simulink model "controladorPaola"  (R2023b)
settings: Solver=ode23t  StartTime=0.0  StopTime=60  MaxStep=1e-3  RelTol=1e-3
values from neighbouring files (symbols this model uses):
  AL = double(subs(A_par))    [ANTImodeloMATEMATICOFINAL.m]
  BL = double(subs(B_par))    [ANTImodeloMATEMATICOFINAL.m]
  Blo = 8.18575752786119e-06    (= 8.18575752786e-06)    [ANTImodeloMATEMATICOFINAL.m]
  Bmo = 2.02156082362446e-07    (= 2.02156082362e-07)    [ANTImodeloMATEMATICOFINAL.m]
  CL = double(subs(C_par))    [ANTImodeloMATEMATICOFINAL.m]
  DL = double(subs(D_par))    [ANTImodeloMATEMATICOFINAL.m]
  do = 0.06862-0.021    (= 0.04762)    [ANTImodeloMATEMATICOFINAL.m]
  go = 9.81    [ANTImodeloMATEMATICOFINAL.m]
  Jlo = 0.00100697016255642    (= 0.00100697016256)    [ANTImodeloMATEMATICOFINAL.m]
  Jmo = 2.08549279330578e-07    (= 2.08549279331e-07)    [ANTImodeloMATEMATICOFINAL.m]
  Kes = K(:,1:n)    [ANTImodeloMATEMATICOFINAL.m]
  Ki = -K(:,n+1:end)    [ANTImodeloMATEMATICOFINAL.m]
  Kio = 0.00119530882984502    (= 0.00119530882985)    [ANTImodeloMATEMATICOFINAL.m]
  Kvo = 0.0035694528924319    (= 0.00356945289243)    [ANTImodeloMATEMATICOFINAL.m]
  Lo = 0.667669785204658    (= 0.667669785205)    [ANTImodeloMATEMATICOFINAL.m]
  mo = 0.17244    [ANTImodeloMATEMATICOFINAL.m]
  no = 120    [ANTImodeloMATEMATICOFINAL.m]
  Ro = 5.15610211779038    (= 5.15610211779)    [ANTImodeloMATEMATICOFINAL.m]
  Tm = 0.03    [ANTImodeloMATEMATICOFINAL.m]
  Vin0 = Ro*X10    (= 0)    [ANTImodeloMATEMATICOFINAL.m]
  X10 = 0    [ANTImodeloMATEMATICOFINAL.m]
  X20 = 0    [ANTImodeloMATEMATICOFINAL.m]
  X30 = 0    [ANTImodeloMATEMATICOFINAL.m]
undefined symbols (not defined in the file or in its folder): Ac_2, Bc_2, Cc_2, Dc_2, L, magnitude, sys_d2
libraries: cstblocks x6, slpidlib x4, simulink x4
(part 1 of 2)
settings Model: Creator=hubertdelgado  LastModifiedBy=electronica
settings DebuggingCC: UnconnectedInputMsg=warning  UnconnectedOutputMsg=warning  UnconnectedLineMsg=warning
settings ModelReferenceCC: EnableRefExpFcnMdlSchedulingChecks=on
settings RTWCC: DLArmComputeVersion=19.05

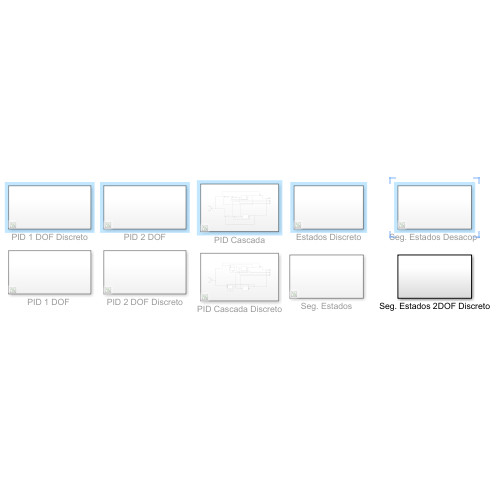
[thumbnail: Simulink's stored preview of the top-level diagram]
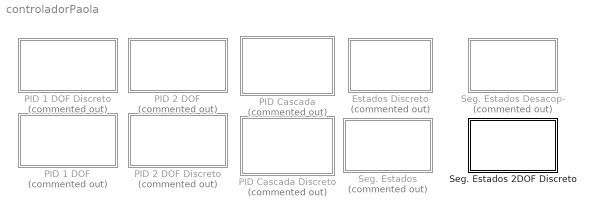
== system controladorPaola ==
  Estados Discreto : Subsystem  Commented=on
  "PID 1 DOF " : Subsystem  Commented=on
  PID 1 DOF Discreto : Subsystem  Commented=on
  PID 2 DOF : Subsystem  Commented=on
  PID 2 DOF Discreto : Subsystem  Commented=on
  PID Cascada : Subsystem  Commented=on
  PID Cascada Discreto : Subsystem  Commented=on
  Seg. Estados : Subsystem  Commented=on
  Seg. Estados 2DOF Discreto : Subsystem
  Seg. Estados Desacop- : Subsystem  Commented=on

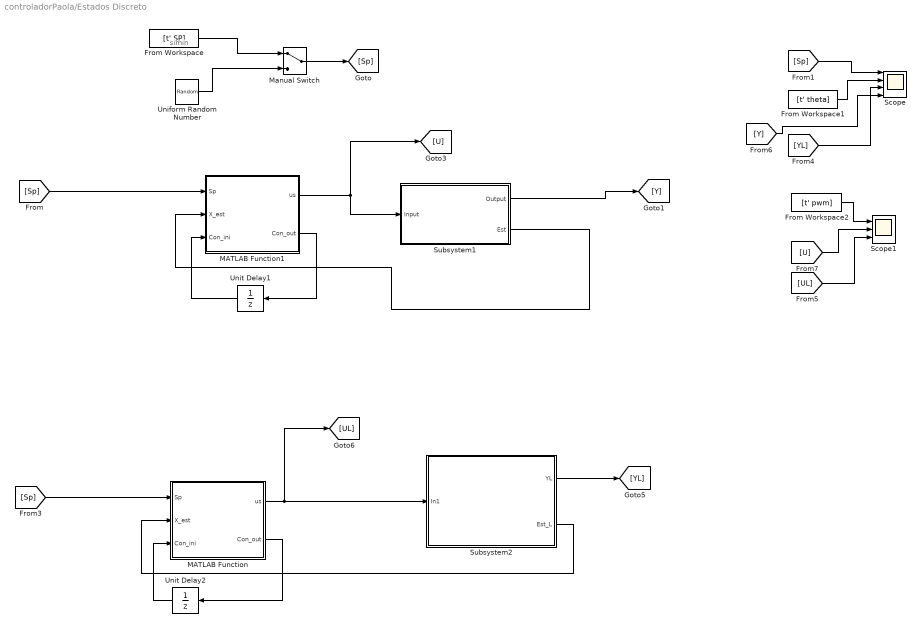
== system controladorPaola/Estados Discreto ==
  note: simin
  From Workspace : FromWorkspace  VariableName=[t' SP]
  From Workspace1 : FromWorkspace  VariableName=[t' theta]
  From Workspace2 : FromWorkspace  VariableName=[t' pwm]
  MATLAB Function : MATLAB Function  TreatAsAtomicUnit=on
  MATLAB Function1 : MATLAB Function  TreatAsAtomicUnit=on
  Manual Switch : ManualSwitch
  Scope : Scope  NumInputPorts=4
  Scope1 : Scope  NumInputPorts=3
  Subsystem1 : Subsystem
  Subsystem2 : Subsystem
  Uniform Random Number : UniformRandomNumber  Minimum=-120*(pi/180)  Maximum=120*(pi/180)  SampleTime=10
  Unit Delay1 : UnitDelay  InitialCondition=zeros(1,2)  SampleTime=Tm  HasFrameUpgradeWarning=on
  Unit Delay2 : UnitDelay  InitialCondition=zeros(1,2)  SampleTime=Tm  HasFrameUpgradeWarning=on
  wires:
  Subsystem1/1(Output) -> [Y]
  MATLAB Function/1(us) -> Subsystem2/1(In1), [UL]
  [Sp] -> MATLAB Function/1(Sp)
  MATLAB Function/2(Con_out) -> Unit Delay2/1
  Unit Delay2/1 -> MATLAB Function/3(Con_ini)
  Subsystem2/2(Est_L) -> MATLAB Function/2(X_est)
  Subsystem2/1(YL) -> [YL]
  Manual Switch/1 -> [Sp]
  [Y] -> Scope/4
  From Workspace2/1 -> Scope1/1
  From Workspace/1 -> Manual Switch/1
  From Workspace1/1 -> Scope/2
  Uniform Random Number/1 -> Manual Switch/2
  [Sp] -> Scope/1
  [UL] -> Scope1/3
  [U] -> Scope1/2
  [YL] -> Scope/3
  Subsystem1/2(Est) -> MATLAB Function1/2(X_est)
  Unit Delay1/1 -> MATLAB Function1/3(Con_ini)
  MATLAB Function1/2(Con_out) -> Unit Delay1/1
  [Sp] -> MATLAB Function1/1(Sp)
  MATLAB Function1/1(us) -> [U], Subsystem1/1(Input)

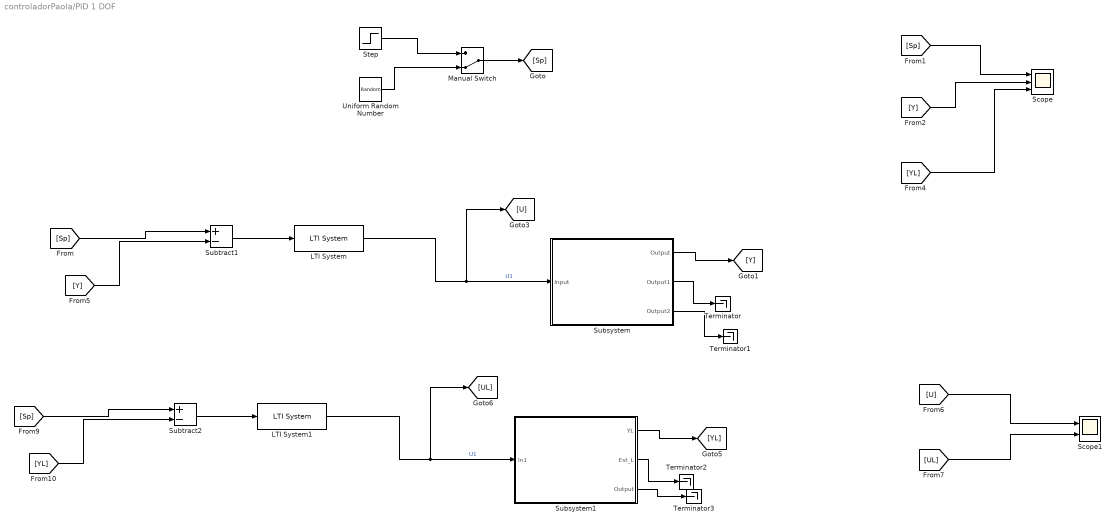
== system controladorPaola/PID 1 DOF  ==
  LTI System : cstblocks/LTI System  sys=Cpids  IC=[]
  LTI System1 : cstblocks/LTI System  sys=Cpids  IC=[]
  Manual Switch : ManualSwitch  CurrentSetting=0
  Scope : Scope  NumInputPorts=3
  Scope1 : Scope  NumInputPorts=2
  Step : Step  Time=0  After=0  SampleTime=0
  Subsystem : Subsystem
  Subsystem1 : Subsystem
  Subtract1 : Sum  Inputs=+-
  Subtract2 : Sum  Inputs=+-
  Terminator{,1..3} (4 alike) : Terminator
  Uniform Random Number : UniformRandomNumber  Minimum=-70*(pi/180)  Maximum=70*(pi/180)  SampleTime=10
  wires:
  Manual Switch/1 -> [Sp]
  Uniform Random Number/1 -> Manual Switch/2
  [U] -> Scope1/1
  [UL] -> Scope1/2
  Step/1 -> Manual Switch/1
  Subtract1/1 -> LTI System/1
  LTI System/1 -> Subsystem/1(Input), [U]  "U1"
  [Sp] -> Subtract1/1
  [Y] -> Subtract1/2
  Subsystem/1(Output) -> [Y]
  Subtract2/1 -> LTI System1/1
  [YL] -> Subtract2/2
  LTI System1/1 -> Subsystem1/1(In1), [UL]  "U1"
  Subsystem1/2(Est_L) -> Terminator2/1
  Subsystem1/1(YL) -> [YL]
  [Sp] -> Subtract2/1
  [Sp] -> Scope/1
  [Y] -> Scope/2
  [YL] -> Scope/3
  Subsystem/2(Output1) -> Terminator/1
  Subsystem/3(Output2) -> Terminator1/1
  Subsystem1/3(Output) -> Terminator3/1

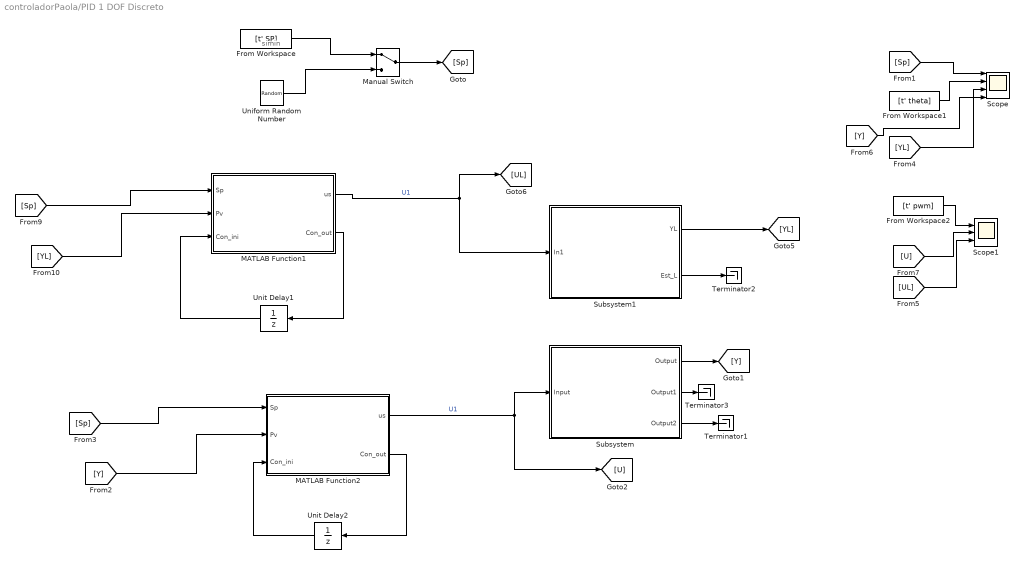
== system controladorPaola/PID 1 DOF Discreto ==
  note: simin
  From Workspace : FromWorkspace  VariableName=[t' SP]
  From Workspace1 : FromWorkspace  VariableName=[t' theta]
  From Workspace2 : FromWorkspace  VariableName=[t' pwm]
  MATLAB Function1 : MATLAB Function  TreatAsAtomicUnit=on
  MATLAB Function2 : MATLAB Function  TreatAsAtomicUnit=on
  Manual Switch : ManualSwitch
  Scope : Scope  NumInputPorts=4
  Scope1 : Scope  NumInputPorts=3
  Subsystem : Subsystem
  Subsystem1 : Subsystem
  Terminator1 : Terminator
  Terminator2 : Terminator
  Terminator3 : Terminator
  Uniform Random Number : UniformRandomNumber  Minimum=-60*(pi/180)  Maximum=60*(pi/180)  SampleTime=10
  Unit Delay1 : UnitDelay  InitialCondition=zeros(4,1)  SampleTime=Tm  HasFrameUpgradeWarning=on
  Unit Delay2 : UnitDelay  InitialCondition=zeros(5,1)  SampleTime=Tm  HasFrameUpgradeWarning=on
  wires:
  Manual Switch/1 -> [Sp]
  Uniform Random Number/1 -> Manual Switch/2
  From Workspace2/1 -> Scope1/1
  [U] -> Scope1/2
  From Workspace/1 -> Manual Switch/1
  [YL] -> MATLAB Function1/2(Pv)
  MATLAB Function1/1(us) -> Subsystem1/1(In1), [UL]  "U1"
  Subsystem1/2(Est_L) -> Terminator2/1
  Subsystem1/1(YL) -> [YL]
  [Sp] -> Scope/1
  From Workspace1/1 -> Scope/2
  [YL] -> Scope/3
  Unit Delay1/1 -> MATLAB Function1/3(Con_ini)
  [Sp] -> MATLAB Function1/1(Sp)
  MATLAB Function1/2(Con_out) -> Unit Delay1/1
  Unit Delay2/1 -> MATLAB Function2/3(Con_ini)
  MATLAB Function2/2(Con_out) -> Unit Delay2/1
  MATLAB Function2/1(us) -> [U], Subsystem/1(Input)  "U1"
  [Sp] -> MATLAB Function2/1(Sp)
  [Y] -> MATLAB Function2/2(Pv)
  Subsystem/1(Output) -> [Y]
  Subsystem/3(Output2) -> Terminator1/1
  Subsystem/2(Output1) -> Terminator3/1
  [UL] -> Scope1/3
  [Y] -> Scope/4

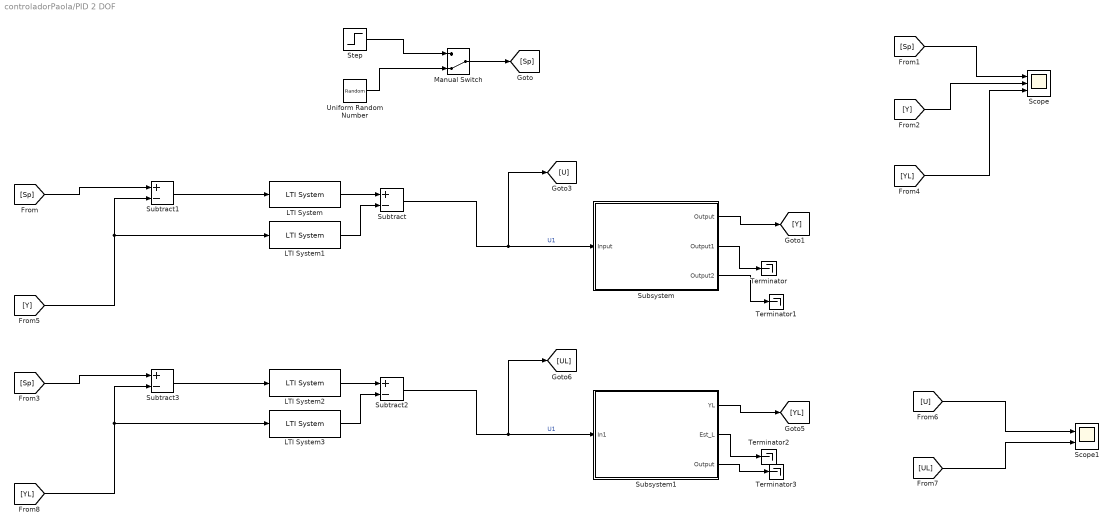
== system controladorPaola/PID 2 DOF ==
  LTI System : cstblocks/LTI System  sys=C1s  IC=[]  PadeOrder=0
  LTI System1 : cstblocks/LTI System  sys=C2s  IC=[]  PadeOrder=0
  LTI System2 : cstblocks/LTI System  sys=C1s  IC=[]  PadeOrder=0
  LTI System3 : cstblocks/LTI System  sys=C2s  IC=[]  PadeOrder=0
  Manual Switch : ManualSwitch  CurrentSetting=0
  Scope : Scope  NumInputPorts=3
  Scope1 : Scope  NumInputPorts=2
  Step : Step  Time=0  After=0  SampleTime=0
  Subsystem : Subsystem
  Subsystem1 : Subsystem
  Subtract{,1..3} (4 alike) : Sum  Inputs=+-
  Terminator{,1..3} (4 alike) : Terminator
  Uniform Random Number : UniformRandomNumber  Minimum=-60*(pi/180)  Maximum=60*(pi/180)  SampleTime=10
  wires:
  LTI System/1 -> Subtract/1
  Subtract1/1 -> LTI System/1
  [Sp] -> Subtract1/1
  [Y] -> LTI System1/1, Subtract1/2
  LTI System1/1 -> Subtract/2
  Subtract2/1 -> Subsystem1/1(In1), [UL]  "U1"
  Subsystem1/3(Output) -> Terminator3/1
  Subtract/1 -> Subsystem/1(Input), [U]  "U1"
  Subsystem1/2(Est_L) -> Terminator2/1
  Subsystem/3(Output2) -> Terminator1/1
  Subsystem1/1(YL) -> [YL]
  Subsystem/2(Output1) -> Terminator/1
  Subsystem/1(Output) -> [Y]
  [Sp] -> Subtract3/1
  LTI System3/1 -> Subtract2/2
  LTI System2/1 -> Subtract2/1
  Subtract3/1 -> LTI System2/1
  [YL] -> LTI System3/1, Subtract3/2
  [UL] -> Scope1/2
  Step/1 -> Manual Switch/1
  Manual Switch/1 -> [Sp]
  [Y] -> Scope/2
  [Sp] -> Scope/1
  [YL] -> Scope/3
  [U] -> Scope1/1
  Uniform Random Number/1 -> Manual Switch/2

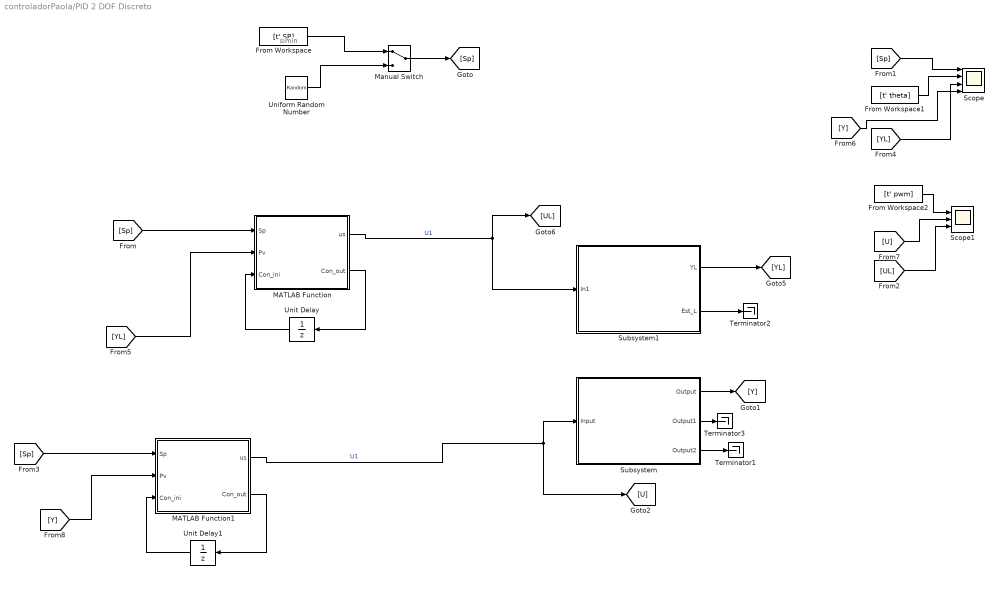
== system controladorPaola/PID 2 DOF Discreto ==
  note: simin
  From Workspace : FromWorkspace  VariableName=[t' SP]
  From Workspace1 : FromWorkspace  VariableName=[t' theta]
  From Workspace2 : FromWorkspace  VariableName=[t' pwm]
  MATLAB Function : MATLAB Function  TreatAsAtomicUnit=on
  MATLAB Function1 : MATLAB Function  TreatAsAtomicUnit=on
  Manual Switch : ManualSwitch
  Scope : Scope  NumInputPorts=4
  Scope1 : Scope  NumInputPorts=3
  Subsystem : Subsystem
  Subsystem1 : Subsystem
  Terminator1 : Terminator
  Terminator2 : Terminator
  Terminator3 : Terminator
  Uniform Random Number : UniformRandomNumber  Minimum=-65*(pi/180)  Maximum=65*(pi/180)  SampleTime=10
  Unit Delay : UnitDelay  InitialCondition=zeros(6,1)  SampleTime=Tm  HasFrameUpgradeWarning=on
  Unit Delay1 : UnitDelay  InitialCondition=zeros(6,1)  SampleTime=Tm  HasFrameUpgradeWarning=on
  wires:
  [Sp] -> MATLAB Function/1(Sp)
  Unit Delay/1 -> MATLAB Function/3(Con_ini)
  MATLAB Function/2(Con_out) -> Unit Delay/1
  From Workspace1/1 -> Scope/2
  [YL] -> Scope/3
  [UL] -> Scope1/3
  [U] -> Scope1/2
  [Sp] -> Scope/1
  Uniform Random Number/1 -> Manual Switch/2
  From Workspace/1 -> Manual Switch/1
  From Workspace2/1 -> Scope1/1
  Manual Switch/1 -> [Sp]
  [Y] -> Scope/4
  Subsystem/2(Output1) -> Terminator3/1
  MATLAB Function/1(us) -> Subsystem1/1(In1), [UL]  "U1"
  Subsystem1/2(Est_L) -> Terminator2/1
  Subsystem1/1(YL) -> [YL]
  Subsystem/3(Output2) -> Terminator1/1
  Subsystem/1(Output) -> [Y]
  MATLAB Function1/1(us) -> [U], Subsystem/1(Input)  "U1"
  [Sp] -> MATLAB Function1/1(Sp)
  Unit Delay1/1 -> MATLAB Function1/3(Con_ini)
  MATLAB Function1/2(Con_out) -> Unit Delay1/1
  [YL] -> MATLAB Function/2(Pv)
  [Y] -> MATLAB Function1/2(Pv)

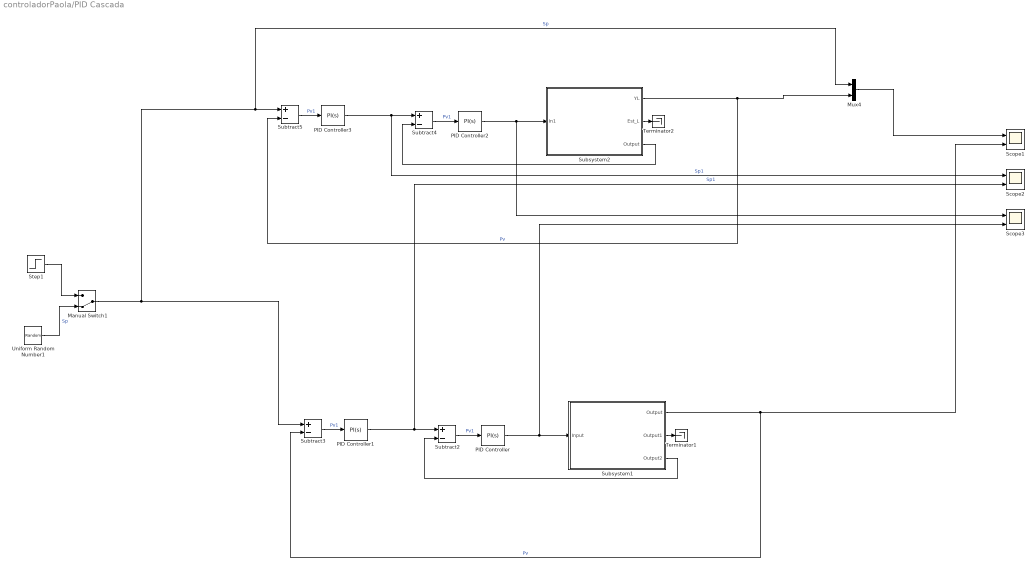
== system controladorPaola/PID Cascada ==
  Manual Switch1 : ManualSwitch  CurrentSetting=0
  Mux4 : Mux  Inputs=2
  PID Controller : slpidlib/PID Controller  Controller=PI  Form=Parallel  TimeDomain=Continuous-time  UseExternalTs=off  SampleTime=-1  IntegratorMethod=Forward Euler  FilterMethod=Forward Euler  ControllerParametersSource=internal  P=0.439531738224972  I=0.0931065859182185  D=35.8399189335653  UseFilter=on  N=15672.9006565225  TunerSelectOption=Transfer Function Based (PID Tuner App)  InitialConditionSource=internal  InitialConditionForIntegrator=0  InitialConditionForFilter=0  DifferentiatorICPrevScaledInput=0  ExternalReset=none  TrackingMode=off  Kt=1  LimitOutput=on  SatLimitsSource=internal  UpperSaturationLimit=100  LowerSaturationLimit=-100  LinearizeAsGain=on  AntiWindupMode=none  Kb=1  POutMin=[]  POutMax=[]  IOutMin=[]  IOutMax=[]  DOutMin=[]  DOutMax=[]  NOutMin=[]  NOutMax=[]  SumOutMin=[]  SumOutMax=[]  SaturationOutMin=[]  SaturationOutMax=[]  PParamMin=[]  PParamMax=[]  IParamMin=[]  IParamMax=[]  DParamMin=[]  DParamMax=[]  NParamMin=[]  NParamMax=[]  KbParamMin=[]  KbParamMax=[]  KtParamMin=[]  KtParamMax=[]  KbOutMin=[]  KbOutMax=[]  KtOutMin=[]  KtOutMax=[]  IntegratorOutMin=[]  IntegratorOutMax=[]  FilterOutMin=[]  FilterOutMax=[]  SumI1OutMin=[]  SumI1OutMax=[]  SumI2OutMin=[]  SumI2OutMax=[]  SumI3OutMin=[]  SumI3OutMax=[]  SumI4OutMin=[]  SumI4OutMax=[]  SumDOutMin=[]  SumDOutMax=[]  DifferentiatorOutMin=[]  DifferentiatorOutMax=[]  FilterDiffOutCoefMin=[]  FilterDiffOutCoefMax=[]  ReciprocalOutMin=[]  ReciprocalOutMax=[]  SumDenOutMin=[]  SumDenOutMax=[]  SumNumOutMin=[]  SumNumOutMax=[]  DivideOutMin=[]  DivideOutMax=[]  UdiffTsProdOutMin=[]  UdiffTsProdOutMax=[]  NTsProdOutMin=[]  NTsProdOutMax=[]  UintegralTsProdOutMin=[]  UintegralTsProdOutMax=[]  UngainTsProdOutMin=[]  UngainTsProdOutMax=[]  IntegratorContinuousStateAttributes=''  IntegratorStateMustResolveToSignalObject=off  IntegratorRTWStateStorageClass=Auto  FilterContinuousStateAttributes=''  FilterStateMustResolveToSignalObject=off  FilterRTWStateStorageClass=Auto  ParallelPVariant=InternalParameters  IdealPVariant=Disabled  IVariant=InternalParameters  DVariant=Disabled  IntegratorVariant=Continuous  SatVariant=Enabled  AWVariant=Passthrough  PCopyVariant=Disabled  TRVariant=Disabled  FdbkBlocksVariant=Forward  IdealPFdbkVariant=Disabled  SatFdbkVariant=Disabled  DerivativeFilterVariant=Disabled  NVariant=Disabled  NCopyVariant=Disabled_SignalSpec  FilterICVariant=Disabled  IntegratorICVariant=InternalICs  ExternalResetVariant=Disabled  TRSumVariant=Passthrough  SumFdbkVariant=Disabled  SumVariant=Sum_PI  TsampFilterVariant=InternalTs  TsampNgainVariant=Passthrough  TsampIntegralVariant=Passthrough  ExternalSaturationOutDataTypeStr=Inherit: Same as second input
  PID Controller1 : slpidlib/PID Controller  Controller=PI  Form=Parallel  TimeDomain=Continuous-time  UseExternalTs=off  SampleTime=-1  IntegratorMethod=Forward Euler  FilterMethod=Forward Euler  ControllerParametersSource=internal  P=0  I=93.1384599522807  D=0.271518816024789  UseFilter=on  N=3961.125137588  TunerSelectOption=Transfer Function Based (PID Tuner App)  InitialConditionSource=internal  InitialConditionForIntegrator=0  InitialConditionForFilter=0  DifferentiatorICPrevScaledInput=0  ExternalReset=none  TrackingMode=off  Kt=1  LimitOutput=on  SatLimitsSource=internal  UpperSaturationLimit=40  LowerSaturationLimit=-40  LinearizeAsGain=on  AntiWindupMode=none  Kb=1  POutMin=[]  POutMax=[]  IOutMin=[]  IOutMax=[]  DOutMin=[]  DOutMax=[]  NOutMin=[]  NOutMax=[]  SumOutMin=[]  SumOutMax=[]  SaturationOutMin=[]  SaturationOutMax=[]  PParamMin=[]  PParamMax=[]  IParamMin=[]  IParamMax=[]  DParamMin=[]  DParamMax=[]  NParamMin=[]  NParamMax=[]  KbParamMin=[]  KbParamMax=[]  KtParamMin=[]  KtParamMax=[]  KbOutMin=[]  KbOutMax=[]  KtOutMin=[]  KtOutMax=[]  IntegratorOutMin=[]  IntegratorOutMax=[]  FilterOutMin=[]  FilterOutMax=[]  SumI1OutMin=[]  SumI1OutMax=[]  SumI2OutMin=[]  SumI2OutMax=[]  SumI3OutMin=[]  SumI3OutMax=[]  SumI4OutMin=[]  SumI4OutMax=[]  SumDOutMin=[]  SumDOutMax=[]  DifferentiatorOutMin=[]  DifferentiatorOutMax=[]  FilterDiffOutCoefMin=[]  FilterDiffOutCoefMax=[]  ReciprocalOutMin=[]  ReciprocalOutMax=[]  SumDenOutMin=[]  SumDenOutMax=[]  SumNumOutMin=[]  SumNumOutMax=[]  DivideOutMin=[]  DivideOutMax=[]  UdiffTsProdOutMin=[]  UdiffTsProdOutMax=[]  NTsProdOutMin=[]  NTsProdOutMax=[]  UintegralTsProdOutMin=[]  UintegralTsProdOutMax=[]  UngainTsProdOutMin=[]  UngainTsProdOutMax=[]  IntegratorContinuousStateAttributes=''  IntegratorStateMustResolveToSignalObject=off  IntegratorRTWStateStorageClass=Auto  FilterContinuousStateAttributes=''  FilterStateMustResolveToSignalObject=off  FilterRTWStateStorageClass=Auto  ParallelPVariant=InternalParameters  IdealPVariant=Disabled  IVariant=InternalParameters  DVariant=Disabled  IntegratorVariant=Continuous  SatVariant=Enabled  AWVariant=Passthrough  PCopyVariant=Disabled  TRVariant=Disabled  FdbkBlocksVariant=Forward  IdealPFdbkVariant=Disabled  SatFdbkVariant=Disabled  DerivativeFilterVariant=Disabled  NVariant=Disabled  NCopyVariant=Disabled_SignalSpec  FilterICVariant=Disabled  IntegratorICVariant=InternalICs  ExternalResetVariant=Disabled  TRSumVariant=Passthrough  SumFdbkVariant=Disabled  SumVariant=Sum_PI  TsampFilterVariant=InternalTs  TsampNgainVariant=Passthrough  TsampIntegralVariant=Passthrough  ExternalSaturationOutDataTypeStr=Inherit: Same as second input
  PID Controller2 : slpidlib/PID Controller  Controller=PI  Form=Parallel  TimeDomain=Continuous-time  UseExternalTs=off  SampleTime=-1  IntegratorMethod=Forward Euler  FilterMethod=Forward Euler  ControllerParametersSource=internal  P=0.439531738224972  I=0.0931065859182185  D=35.8399189335653  UseFilter=on  N=15672.9006565225  TunerSelectOption=Transfer Function Based (PID Tuner App)  InitialConditionSource=internal  InitialConditionForIntegrator=0  InitialConditionForFilter=0  DifferentiatorICPrevScaledInput=0  ExternalReset=none  TrackingMode=off  Kt=1  LimitOutput=on  SatLimitsSource=internal  UpperSaturationLimit=100  LowerSaturationLimit=-100  LinearizeAsGain=on  AntiWindupMode=none  Kb=1  POutMin=[]  POutMax=[]  IOutMin=[]  IOutMax=[]  DOutMin=[]  DOutMax=[]  NOutMin=[]  NOutMax=[]  SumOutMin=[]  SumOutMax=[]  SaturationOutMin=[]  SaturationOutMax=[]  PParamMin=[]  PParamMax=[]  IParamMin=[]  IParamMax=[]  DParamMin=[]  DParamMax=[]  NParamMin=[]  NParamMax=[]  KbParamMin=[]  KbParamMax=[]  KtParamMin=[]  KtParamMax=[]  KbOutMin=[]  KbOutMax=[]  KtOutMin=[]  KtOutMax=[]  IntegratorOutMin=[]  IntegratorOutMax=[]  FilterOutMin=[]  FilterOutMax=[]  SumI1OutMin=[]  SumI1OutMax=[]  SumI2OutMin=[]  SumI2OutMax=[]  SumI3OutMin=[]  SumI3OutMax=[]  SumI4OutMin=[]  SumI4OutMax=[]  SumDOutMin=[]  SumDOutMax=[]  DifferentiatorOutMin=[]  DifferentiatorOutMax=[]  FilterDiffOutCoefMin=[]  FilterDiffOutCoefMax=[]  ReciprocalOutMin=[]  ReciprocalOutMax=[]  SumDenOutMin=[]  SumDenOutMax=[]  SumNumOutMin=[]  SumNumOutMax=[]  DivideOutMin=[]  DivideOutMax=[]  UdiffTsProdOutMin=[]  UdiffTsProdOutMax=[]  NTsProdOutMin=[]  NTsProdOutMax=[]  UintegralTsProdOutMin=[]  UintegralTsProdOutMax=[]  UngainTsProdOutMin=[]  UngainTsProdOutMax=[]  IntegratorContinuousStateAttributes=''  IntegratorStateMustResolveToSignalObject=off  IntegratorRTWStateStorageClass=Auto  FilterContinuousStateAttributes=''  FilterStateMustResolveToSignalObject=off  FilterRTWStateStorageClass=Auto  ParallelPVariant=InternalParameters  IdealPVariant=Disabled  IVariant=InternalParameters  DVariant=Disabled  IntegratorVariant=Continuous  SatVariant=Enabled  AWVariant=Passthrough  PCopyVariant=Disabled  TRVariant=Disabled  FdbkBlocksVariant=Forward  IdealPFdbkVariant=Disabled  SatFdbkVariant=Disabled  DerivativeFilterVariant=Disabled  NVariant=Disabled  NCopyVariant=Disabled_SignalSpec  FilterICVariant=Disabled  IntegratorICVariant=InternalICs  ExternalResetVariant=Disabled  TRSumVariant=Passthrough  SumFdbkVariant=Disabled  SumVariant=Sum_PI  TsampFilterVariant=InternalTs  TsampNgainVariant=Passthrough  TsampIntegralVariant=Passthrough  ExternalSaturationOutDataTypeStr=Inherit: Same as second input
  PID Controller3 : slpidlib/PID Controller  Controller=PI  Form=Parallel  TimeDomain=Continuous-time  UseExternalTs=off  SampleTime=-1  IntegratorMethod=Forward Euler  FilterMethod=Forward Euler  ControllerParametersSource=internal  P=0  I=93.1384599522807  D=0.271518816024789  UseFilter=on  N=3961.125137588  TunerSelectOption=Transfer Function Based (PID Tuner App)  InitialConditionSource=internal  InitialConditionForIntegrator=0  InitialConditionForFilter=0  DifferentiatorICPrevScaledInput=0  ExternalReset=none  TrackingMode=off  Kt=1  LimitOutput=on  SatLimitsSource=internal  UpperSaturationLimit=40  LowerSaturationLimit=-40  LinearizeAsGain=on  AntiWindupMode=none  Kb=1  POutMin=[]  POutMax=[]  IOutMin=[]  IOutMax=[]  DOutMin=[]  DOutMax=[]  NOutMin=[]  NOutMax=[]  SumOutMin=[]  SumOutMax=[]  SaturationOutMin=[]  SaturationOutMax=[]  PParamMin=[]  PParamMax=[]  IParamMin=[]  IParamMax=[]  DParamMin=[]  DParamMax=[]  NParamMin=[]  NParamMax=[]  KbParamMin=[]  KbParamMax=[]  KtParamMin=[]  KtParamMax=[]  KbOutMin=[]  KbOutMax=[]  KtOutMin=[]  KtOutMax=[]  IntegratorOutMin=[]  IntegratorOutMax=[]  FilterOutMin=[]  FilterOutMax=[]  SumI1OutMin=[]  SumI1OutMax=[]  SumI2OutMin=[]  SumI2OutMax=[]  SumI3OutMin=[]  SumI3OutMax=[]  SumI4OutMin=[]  SumI4OutMax=[]  SumDOutMin=[]  SumDOutMax=[]  DifferentiatorOutMin=[]  DifferentiatorOutMax=[]  FilterDiffOutCoefMin=[]  FilterDiffOutCoefMax=[]  ReciprocalOutMin=[]  ReciprocalOutMax=[]  SumDenOutMin=[]  SumDenOutMax=[]  SumNumOutMin=[]  SumNumOutMax=[]  DivideOutMin=[]  DivideOutMax=[]  UdiffTsProdOutMin=[]  UdiffTsProdOutMax=[]  NTsProdOutMin=[]  NTsProdOutMax=[]  UintegralTsProdOutMin=[]  UintegralTsProdOutMax=[]  UngainTsProdOutMin=[]  UngainTsProdOutMax=[]  IntegratorContinuousStateAttributes=''  IntegratorStateMustResolveToSignalObject=off  IntegratorRTWStateStorageClass=Auto  FilterContinuousStateAttributes=''  FilterStateMustResolveToSignalObject=off  FilterRTWStateStorageClass=Auto  ParallelPVariant=InternalParameters  IdealPVariant=Disabled  IVariant=InternalParameters  DVariant=Disabled  IntegratorVariant=Continuous  SatVariant=Enabled  AWVariant=Passthrough  PCopyVariant=Disabled  TRVariant=Disabled  FdbkBlocksVariant=Forward  IdealPFdbkVariant=Disabled  SatFdbkVariant=Disabled  DerivativeFilterVariant=Disabled  NVariant=Disabled  NCopyVariant=Disabled_SignalSpec  FilterICVariant=Disabled  IntegratorICVariant=InternalICs  ExternalResetVariant=Disabled  TRSumVariant=Passthrough  SumFdbkVariant=Disabled  SumVariant=Sum_PI  TsampFilterVariant=InternalTs  TsampNgainVariant=Passthrough  TsampIntegralVariant=Passthrough  ExternalSaturationOutDataTypeStr=Inherit: Same as second input
  Scope1 : Scope  NumInputPorts=2
  Scope2 : Scope  NumInputPorts=2
  Scope3 : Scope  NumInputPorts=2
  Step1 : Step  Time=0  After=2*pi/180  SampleTime=0
  Subsystem1 : Subsystem
  Subsystem2 : Subsystem
  Subtract{2..5} (4 alike) : Sum  Inputs=+-
  Terminator1 : Terminator
  Terminator2 : Terminator
  Uniform Random Number1 : UniformRandomNumber  Minimum=-30*(pi/180)  Maximum=30*(pi/180)  SampleTime=15
  wires:
  Step1/1 -> Manual Switch1/1
  Subsystem1/1(Output) -> Subtract3/2, Scope1/2  "Pv"
  Uniform Random Number1/1 -> Manual Switch1/2  "Sp"
  Subsystem1/2(Output1) -> Terminator1/1
  PID Controller/1 -> Scope3/2, Subsystem1/1(Input)
  Subtract2/1 -> PID Controller/1  "Pv1"
  PID Controller1/1 -> Scope2/2, Subtract2/1  "Sp1"
  Subsystem1/3(Output2) -> Subtract2/2
  Subtract3/1 -> PID Controller1/1  "Pv1"
  Subtract5/1 -> PID Controller3/1  "Pv1"
  Mux4/1 -> Scope1/1
  Subtract4/1 -> PID Controller2/1  "Pv1"
  Subsystem2/2(Est_L) -> Terminator2/1
  Subsystem2/3(Output) -> Subtract4/2
  PID Controller2/1 -> Scope3/1, Subsystem2/1(In1)
  PID Controller3/1 -> Scope2/1, Subtract4/1  "Sp1"
  Subsystem2/1(YL) -> Subtract5/2, Mux4/2  "Pv"
  Manual Switch1/1 -> Mux4/1, Subtract5/1, Subtract3/1  "Sp"

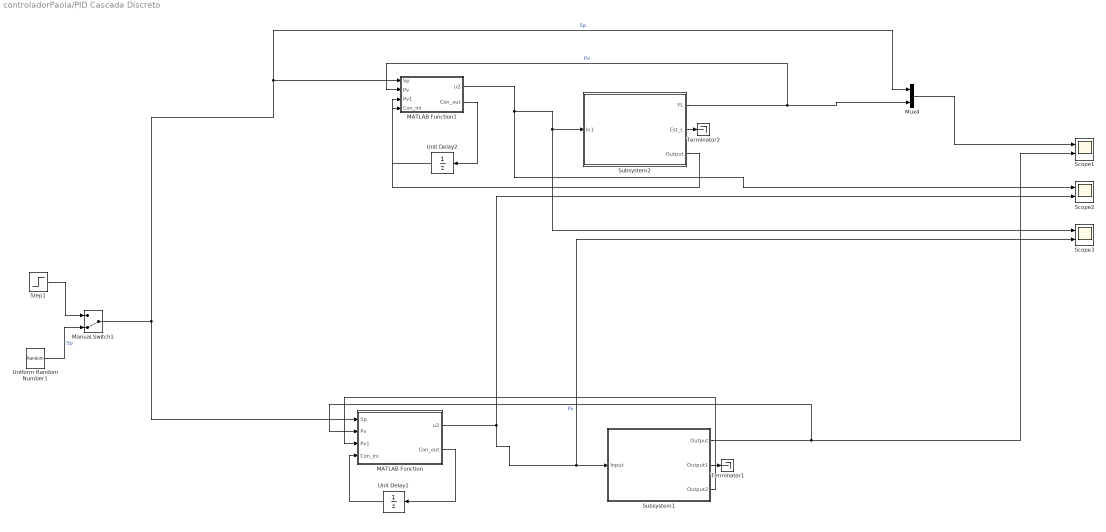
== system controladorPaola/PID Cascada Discreto ==
  MATLAB Function : MATLAB Function  TreatAsAtomicUnit=on
  MATLAB Function1 : MATLAB Function  TreatAsAtomicUnit=on
  Manual Switch1 : ManualSwitch  CurrentSetting=0
  Mux4 : Mux  Inputs=2
  Scope1 : Scope  NumInputPorts=2
  Scope2 : Scope  NumInputPorts=2
  Scope3 : Scope  NumInputPorts=2
  Step1 : Step  Time=0  After=0*pi/180  SampleTime=0
  Subsystem1 : Subsystem
  Subsystem2 : Subsystem
  Terminator1 : Terminator
  Terminator2 : Terminator
  Uniform Random Number1 : UniformRandomNumber  Minimum=-10*(pi/180)  Maximum=10*(pi/180)  SampleTime=15
  Unit Delay1 : UnitDelay  InitialCondition=zeros(4,1)  SampleTime=Tm  HasFrameUpgradeWarning=on
  Unit Delay2 : UnitDelay  InitialCondition=zeros(4,1)  SampleTime=Tm  HasFrameUpgradeWarning=on
  wires:
  Step1/1 -> Manual Switch1/1
  Subsystem1/1(Output) -> MATLAB Function/2(Pv), Scope1/2  "Pv"
  Uniform Random Number1/1 -> Manual Switch1/2  "Sp"
  Subsystem1/2(Output1) -> Terminator1/1
  MATLAB Function/1(u2) -> Scope3/2, Subsystem1/1(Input), Scope2/2
  Mux4/1 -> Scope1/1
  Subsystem2/2(Est_L) -> Terminator2/1
  MATLAB Function1/1(u2) -> Scope2/1, Scope3/1, Subsystem2/1(In1)
  Subsystem2/1(YL) -> MATLAB Function1/2(Pv), Mux4/2  "Pv"
  Subsystem2/3(Output) -> MATLAB Function1/3(Pv1)
  MATLAB Function1/2(Con_out) -> Unit Delay2/1
  MATLAB Function/2(Con_out) -> Unit Delay1/1
  Manual Switch1/1 -> MATLAB Function/1(Sp), Mux4/1, MATLAB Function1/1(Sp)  "Sp"
  Subsystem1/3(Output2) -> MATLAB Function/3(Pv1)
  Unit Delay1/1 -> MATLAB Function/4(Con_ini)
  Unit Delay2/1 -> MATLAB Function1/4(Con_ini)

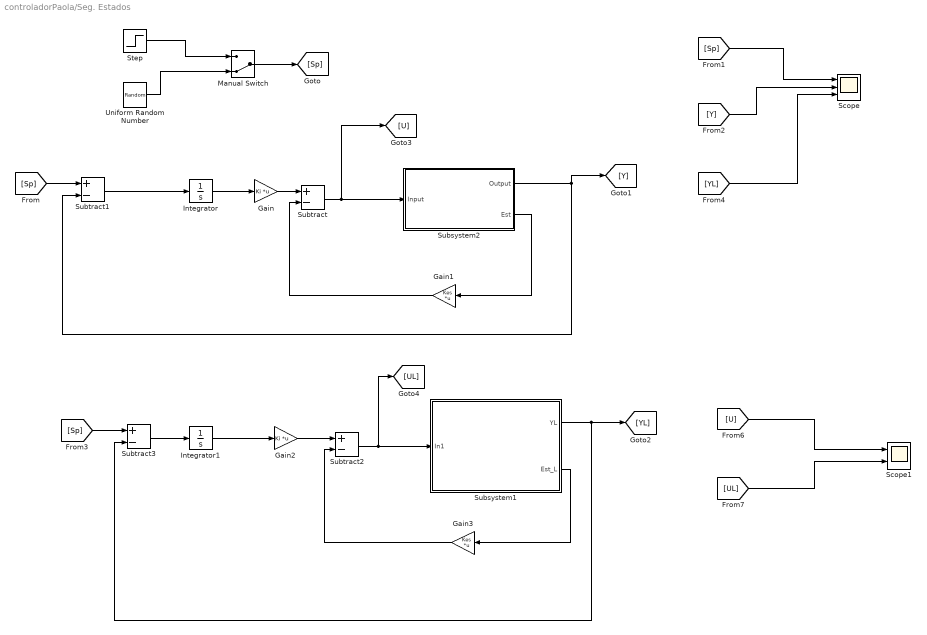
== system controladorPaola/Seg. Estados ==
  Gain : Gain  Gain=Ki  Multiplication=Matrix(K*u)
  Gain1 : Gain  Gain=Kes  Multiplication=Matrix(K*u)
  Gain2 : Gain  Gain=Ki  Multiplication=Matrix(K*u)
  Gain3 : Gain  Gain=Kes  Multiplication=Matrix(K*u)
  Integrator : Integrator
  Integrator1 : Integrator
  Manual Switch : ManualSwitch  CurrentSetting=0
  Scope : Scope  NumInputPorts=3
  Scope1 : Scope  NumInputPorts=2
  Step : Step  Time=0  After=0  SampleTime=0
  Subsystem1 : Subsystem
  Subsystem2 : Subsystem
  Subtract{,1..3} (4 alike) : Sum  Inputs=+-
  Uniform Random Number : UniformRandomNumber  Minimum=-120*(pi/180)  Maximum=120*(pi/180)  SampleTime=10
  wires:
  Subsystem2/1(Output) -> Subtract1/2, [Y]
  Subsystem2/2(Est) -> Gain1/1
  Subtract/1 -> Subsystem2/1(Input), [U]
  Gain1/1 -> Subtract/2
  Subtract2/1 -> [UL], Subsystem1/1(In1)
  Gain/1 -> Subtract/1
  [Sp] -> Subtract1/1
  [Sp] -> Subtract3/1
  Gain2/1 -> Subtract2/1
  Subsystem1/1(YL) -> [YL], Subtract3/2
  Subsystem1/2(Est_L) -> Gain3/1
  Gain3/1 -> Subtract2/2
  Integrator/1 -> Gain/1
  Subtract1/1 -> Integrator/1
  Integrator1/1 -> Gain2/1
  Subtract3/1 -> Integrator1/1
  [UL] -> Scope1/2
  Step/1 -> Manual Switch/1
  Manual Switch/1 -> [Sp]
  [Y] -> Scope/2
  [Sp] -> Scope/1
  [YL] -> Scope/3
  [U] -> Scope1/1
  Uniform Random Number/1 -> Manual Switch/2

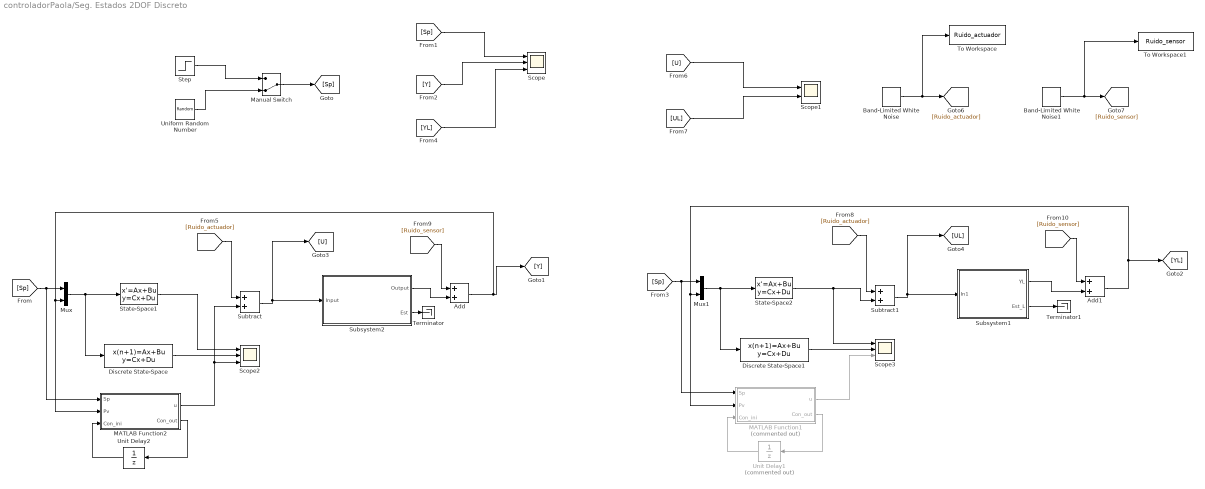
== system controladorPaola/Seg. Estados 2DOF Discreto ==
  Add : Sum
  Add1 : Sum
  Band-Limited White Noise : simulink/Sources/Band-Limited White Noise  Cov=[1e-10]  Ts=0.001  seed=[23341]
  Band-Limited White Noise1 : simulink/Sources/Band-Limited White Noise  Cov=[1e-10]  Ts=0.001  seed=[23341]
  Discrete State-Space : DiscreteStateSpace  A=sys_d2.a  B=sys_d2.b  C=sys_d2.c  D=sys_d2.d  SampleTime=Tm
  Discrete State-Space1 : DiscreteStateSpace  A=sys_d2.a  B=sys_d2.b  C=sys_d2.c  D=sys_d2.d  SampleTime=Tm
  MATLAB Function1 : MATLAB Function  Commented=on  TreatAsAtomicUnit=on
  MATLAB Function2 : MATLAB Function  TreatAsAtomicUnit=on
  Manual Switch : ManualSwitch  CurrentSetting=0
  Mux : Mux  Inputs=2
  Mux1 : Mux  Inputs=2
  Scope : Scope  NumInputPorts=3
  Scope1 : Scope  NumInputPorts=2
  Scope2 : Scope  NumInputPorts=3
  Scope3 : Scope  NumInputPorts=3
  State-Space1 : StateSpace  A=Ac_2  B=Bc_2  C=Cc_2  D=Dc_2  InitialCondition=0
  State-Space2 : StateSpace  A=Ac_2  B=Bc_2  C=Cc_2  D=Dc_2  InitialCondition=0
  Step : Step  Time=0  After=0  SampleTime=0
  Subsystem1 : Subsystem
  Subsystem2 : Subsystem
  Subtract : Sum
  Subtract1 : Sum
  Terminator : Terminator
  Terminator1 : Terminator
  To Workspace : ToWorkspace  VariableName=Ruido_actuador  SampleTime=-1
  To Workspace1 : ToWorkspace  VariableName=Ruido_sensor  SampleTime=-1
  Uniform Random Number : UniformRandomNumber  Minimum=-65*(pi/180)  Maximum=65*(pi/180)  SampleTime=10
  Unit Delay1 : UnitDelay  Commented=on  InitialCondition=zeros(8,1)  SampleTime=Tm  HasFrameUpgradeWarning=on
  Unit Delay2 : UnitDelay  InitialCondition=zeros(5,1)  SampleTime=Tm  HasFrameUpgradeWarning=on
  wires:
  [Sp] -> MATLAB Function2/1(Sp), Mux/1
  Band-Limited White Noise/1 -> To Workspace/1, [Ruido_actuador]
  Band-Limited White Noise1/1 -> To Workspace1/1, [Ruido_sensor]
  [UL] -> Scope1/2
  Uniform Random Number/1 -> Manual Switch/2
  [Sp] -> Scope/1
  [U] -> Scope1/1
  Step/1 -> Manual Switch/1
  Manual Switch/1 -> [Sp]
  [YL] -> Scope/3
  [Y] -> Scope/2
  Subtract/1 -> Subsystem2/1(Input), [U]
  State-Space1/1 -> Scope2/1
  [Ruido_actuador] -> Subtract/1
  Add/1 -> MATLAB Function2/2(Pv), Mux/2, [Y]
  Subsystem2/1(Output) -> Add/2
  [Ruido_sensor] -> Add/1
  Subsystem2/2(Est) -> Terminator/1
  Mux/1 -> Discrete State-Space/1, State-Space1/1
  Discrete State-Space/1 -> Scope2/2
  MATLAB Function2/2(Con_out) -> Unit Delay2/1
  Unit Delay2/1 -> MATLAB Function2/3(Con_ini)
  MATLAB Function2/1(u) -> Subtract/2, Scope2/3
  [Sp] -> MATLAB Function1/1(Sp), Mux1/1
  Subsystem1/2(Est_L) -> Terminator1/1
  MATLAB Function1/1(u) -> Scope3/3
  [Ruido_sensor] -> Add1/1
  Subsystem1/1(YL) -> Add1/2
  Add1/1 -> MATLAB Function1/2(Pv), Mux1/2, [YL]
  Subtract1/1 -> Subsystem1/1(In1), [UL]
  [Ruido_actuador] -> Subtract1/1
  Discrete State-Space1/1 -> Scope3/2
  Unit Delay1/1 -> MATLAB Function1/3(Con_ini)
  Mux1/1 -> Discrete State-Space1/1, State-Space2/1
  State-Space2/1 -> Scope3/1, Subtract1/2
  MATLAB Function1/2(Con_out) -> Unit Delay1/1

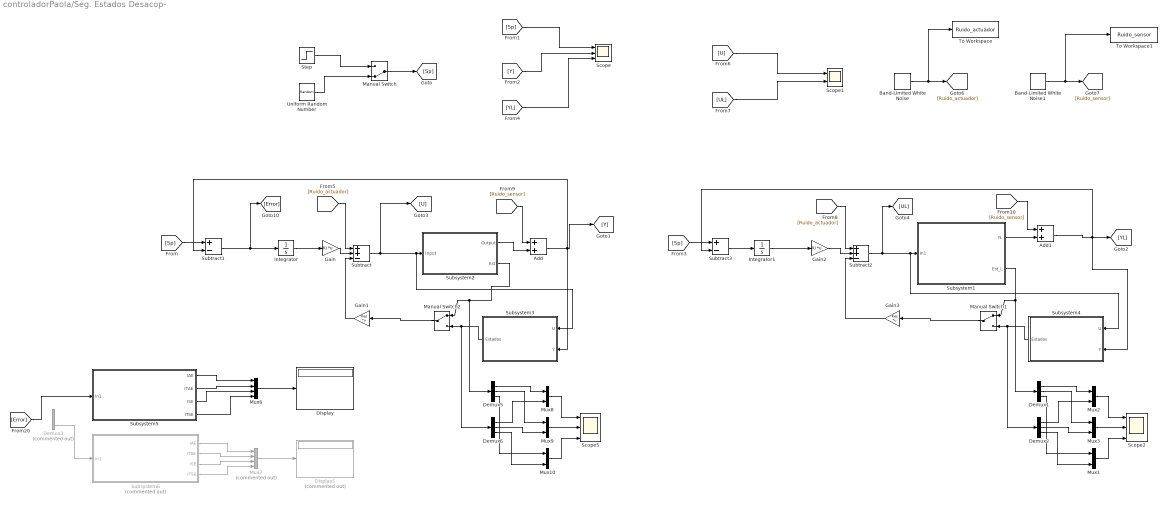
== system controladorPaola/Seg. Estados Desacop- ==
  Add : Sum
  Add1 : Sum
  Band-Limited White Noise : simulink/Sources/Band-Limited White Noise  Cov=[1e-10]  Ts=0.001  seed=[23341]
  Band-Limited White Noise1 : simulink/Sources/Band-Limited White Noise  Cov=[1e-10]  Ts=0.001  seed=[23341]
  Demux{1..2,5..6} (4 alike) : Demux  Outputs=3
  Demux3 : Demux  Commented=on  Outputs=2
  Display : Display
  Display1 : Display  Commented=on
  Gain : Gain  Gain=Ki  Multiplication=Matrix(K*u)
  Gain1 : Gain  Gain=Kes  Multiplication=Matrix(K*u)
  Gain2 : Gain  Gain=Ki  Multiplication=Matrix(K*u)
  Gain3 : Gain  Gain=Kes  Multiplication=Matrix(K*u)
  Integrator : Integrator
  Integrator1 : Integrator
  Manual Switch : ManualSwitch  CurrentSetting=0
  Manual Switch1 : ManualSwitch
  Manual Switch2 : ManualSwitch
  Mux{1..3,8..10} (6 alike) : Mux  Inputs=2
  Mux6 : Mux
  Mux7 : Mux  Commented=on
  Scope : Scope  NumInputPorts=3
  Scope1 : Scope  NumInputPorts=2
  Scope2 : Scope  NumInputPorts=3
  Scope5 : Scope  NumInputPorts=3
  Step : Step  Time=0  After=0  SampleTime=0
  Subsystem1 : Subsystem
  Subsystem2 : Subsystem
  Subsystem3 : Subsystem
  Subsystem4 : Subsystem
  Subsystem5 : Subsystem
  Subsystem6 : Subsystem  Commented=on
  Subtract : Sum  Inputs=++-
  Subtract1 : Sum  Inputs=+-
  Subtract2 : Sum  Inputs=++-
  Subtract3 : Sum  Inputs=+-
  To Workspace : ToWorkspace  VariableName=Ruido_actuador  SampleTime=-1
  To Workspace1 : ToWorkspace  VariableName=Ruido_sensor  SampleTime=-1
  Uniform Random Number : UniformRandomNumber  Minimum=-65*(pi/180)  Maximum=65*(pi/180)  SampleTime=10
  wires:
  [Sp] -> Subtract1/1
  [Sp] -> Subtract3/1
  Integrator/1 -> Gain/1
  Integrator1/1 -> Gain2/1
  Subtract3/1 -> Integrator1/1
  Band-Limited White Noise/1 -> To Workspace/1, [Ruido_actuador]
  Band-Limited White Noise1/1 -> To Workspace1/1, [Ruido_sensor]
  [UL] -> Scope1/2
  Uniform Random Number/1 -> Manual Switch/2
  [Sp] -> Scope/1
  [U] -> Scope1/1
  Step/1 -> Manual Switch/1
  Manual Switch/1 -> [Sp]
  [YL] -> Scope/3
  [Y] -> Scope/2
  Subtract/1 -> Subsystem3/1(U), Subsystem2/1(Input), [U]
  Mux10/1 -> Scope5/3
  Demux6/1 -> Mux8/2
  Demux5/2 -> Mux9/1
  Mux8/1 -> Scope5/1
  Demux6/3 -> Mux10/2
  Demux6/2 -> Mux9/2
  Demux5/3 -> Mux10/1
  Mux9/1 -> Scope5/2
  Subsystem3/1(Estados) -> Demux6/1, Manual Switch2/2
  Demux5/1 -> Mux8/1
  Subsystem2/2(Est) -> Demux5/1, Manual Switch2/1
  Manual Switch2/1 -> Gain1/1
  Subtract2/1 -> [UL], Subsystem4/1(U), Subsystem1/1(In1)
  Mux1/1 -> Scope2/3
  Demux2/1 -> Mux2/2
  Demux1/2 -> Mux3/1
  Mux2/1 -> Scope2/1
  Demux2/3 -> Mux1/2
  Demux2/2 -> Mux3/2
  Demux1/3 -> Mux1/1
  Mux3/1 -> Scope2/2
  Subsystem4/1(Estados) -> Demux2/1, Manual Switch1/2
  Demux1/1 -> Mux2/1
  Subsystem1/2(Est_L) -> Demux1/1, Manual Switch1/1
  Manual Switch1/1 -> Gain3/1
  Subtract1/1 -> [Error], Integrator/1
  Subsystem5/2(ITAE) -> Mux6/2
  Subsystem5/4(ITSE) -> Mux6/4
  Subsystem5/3(ISE) -> Mux6/3
  Subsystem5/1(IAE) -> Mux6/1
  Mux7/1 -> Display1/1
  Subsystem6/1(IAE) -> Mux7/1
  Subsystem6/4(ITSE) -> Mux7/4
  Mux6/1 -> Display/1
  Demux3/2 -> Subsystem6/1(In1)
  Subsystem6/3(ISE) -> Mux7/3
  Subsystem6/2(ITAE) -> Mux7/2
  [Error] -> Subsystem5/1(In1)
  Gain/1 -> Subtract/2
  Gain1/1 -> Subtract/3
  [Ruido_actuador] -> Subtract/1
  Gain2/1 -> Subtract2/2
  Gain3/1 -> Subtract2/3
  [Ruido_actuador] -> Subtract2/1
  Add/1 -> Subtract1/2, Subsystem3/2(Y), [Y]
  Subsystem2/1(Output) -> Add/2
  [Ruido_sensor] -> Add/1
  Subsystem1/1(YL) -> Add1/2
  Add1/1 -> Subsystem4/2(Y), Subtract3/2, [YL]
  [Ruido_sensor] -> Add1/1

== system controladorPaola/Estados Discreto/Subsystem1 ==
  Input : Inport
  Add : Sum
  Constant : Constant  Value=[Ro,Lo,Kio, Kvo, Jmo, Jlo, Bmo, Blo, no, go, do, mo]
  Constant1 : Constant  Value=Vin0
  Constant2 : Constant  Value=[X10; X20]
  Gain1 : Gain  Gain=CL  Multiplication=Matrix(K*u)
  Integrator : Integrator  InitialCondition=[X10; X20]
  MATLAB Function : MATLAB Function  TreatAsAtomicUnit=on
  Subtract1 : Sum  Inputs=+-
  Output : Outport
  Est : Outport  Port=2
  wires:
  Add/1 -> MATLAB Function/2(PWM)
  Constant2/1 -> Subtract1/2
  Constant1/1 -> Add/1
  Input/1 -> Add/2
  MATLAB Function/1(dx) -> Integrator/1
  Constant/1 -> MATLAB Function/3(parametros)
  Integrator/1 -> Subtract1/1, MATLAB Function/1(x)
  Subtract1/1 -> Est/1, Gain1/1
  Gain1/1 -> Output/1

== system controladorPaola/Estados Discreto/Subsystem2 ==
  In1 : Inport
  Add : Sum
  Add1 : Sum
  Gain : Gain  Gain=CL  Multiplication=Matrix(K*u)
  Gain1 : Gain  Gain=AL  Multiplication=Matrix(K*u)
  Gain2 : Gain  Gain=DL  Multiplication=Matrix(K*u)
  Gain3 : Gain  Gain=BL  Multiplication=Matrix(K*u)
  Integrator : Integrator
  YL : Outport
  Est_L : Outport  Port=2
  wires:
  Gain/1 -> Add/2
  Integrator/1 -> Gain/1, Est_L/1, Gain1/1
  Add1/1 -> Integrator/1
  Gain1/1 -> Add1/2
  Gain2/1 -> Add/1
  Gain3/1 -> Add1/1
  Add/1 -> YL/1
  In1/1 -> Gain2/1, Gain3/1

== system controladorPaola/PID 1 DOF /Subsystem ==
  Input : Inport
  Add : Sum
  Constant : Constant  Value=[Ro, Lo, Kio, Kvo, Jmo, Jlo, Bmo, Blo, no, go, do, mo]
  Constant1 : Constant  Value=Vin0
  Constant2 : Constant  Value=[X10; X20; X30]
  Demux : Demux  Outputs=2
  Gain : Gain  Gain=DL  Multiplication=Matrix(K*u)
  Gain1 : Gain  Gain=CL  Multiplication=Matrix(K*u)
  Integrator : Integrator  InitialCondition=[X10; X20; X30]
  MATLAB Function : MATLAB Function  TreatAsAtomicUnit=on
  Subtract : Sum
  Subtract1 : Sum  Inputs=+-
  Output : Outport
  Output1 : Outport  Port=2
  Output2 : Outport  Port=3
  wires:
  Integrator/1 -> Subtract1/1, MATLAB Function/1(x)
  Add/1 -> MATLAB Function/2(PWM)
  Subtract1/1 -> Output1/1, Gain1/1
  MATLAB Function/1(dx) -> Integrator/1
  Constant1/1 -> Add/1
  Constant2/1 -> Subtract1/2
  Constant/1 -> MATLAB Function/3(parametros)
  Gain1/1 -> Subtract/1
  Gain/1 -> Subtract/2
  Input/1 -> Gain/1, Add/2
  Subtract/1 -> Demux/1
  Demux/1 -> Output/1
  Demux/2 -> Output2/1

== system controladorPaola/PID 1 DOF /Subsystem1 ==
  In1 : Inport
  Add : Sum
  Add1 : Sum
  Demux : Demux  Outputs=2
  Gain : Gain  Gain=CL  Multiplication=Matrix(K*u)
  Gain1 : Gain  Gain=AL  Multiplication=Matrix(K*u)
  Gain2 : Gain  Gain=DL  Multiplication=Matrix(K*u)
  Gain3 : Gain  Gain=BL  Multiplication=Matrix(K*u)
  Integrator : Integrator
  YL : Outport
  Est_L : Outport  Port=2
  Output : Outport  Port=3
  wires:
  Gain/1 -> Add/2
  Integrator/1 -> Gain/1, Est_L/1, Gain1/1
  Add1/1 -> Integrator/1
  Gain1/1 -> Add1/2
  Gain2/1 -> Add/1
  Gain3/1 -> Add1/1
  In1/1 -> Gain2/1, Gain3/1
  Add/1 -> Demux/1
  Demux/1 -> YL/1
  Demux/2 -> Output/1

== system controladorPaola/PID 1 DOF Discreto/Subsystem ==
  Input : Inport
  Add : Sum
  Constant : Constant  Value=[Ro, Lo, Kio, Kvo, Jmo, Jlo, Bmo, Blo, no, go, do, mo]
  Constant1 : Constant  Value=Vin0
  Constant2 : Constant  Value=[X10; X20; X30]
  Demux : Demux  Outputs=2
  Gain : Gain  Gain=DL  Multiplication=Matrix(K*u)
  Gain1 : Gain  Gain=CL  Multiplication=Matrix(K*u)
  Integrator : Integrator  InitialCondition=[X10; X20; X30]
  MATLAB Function : MATLAB Function  TreatAsAtomicUnit=on
  Subtract : Sum
  Subtract1 : Sum  Inputs=+-
  Output : Outport
  Output1 : Outport  Port=2
  Output2 : Outport  Port=3
  wires:
  Integrator/1 -> Subtract1/1, MATLAB Function/1(x)
  Add/1 -> MATLAB Function/2(PWM)
  Subtract1/1 -> Output1/1, Gain1/1
  MATLAB Function/1(dx) -> Integrator/1
  Constant1/1 -> Add/1
  Constant2/1 -> Subtract1/2
  Constant/1 -> MATLAB Function/3(parametros)
  Gain1/1 -> Subtract/1
  Gain/1 -> Subtract/2
  Input/1 -> Gain/1, Add/2
  Subtract/1 -> Demux/1
  Demux/1 -> Output/1
  Demux/2 -> Output2/1

== system controladorPaola/PID 1 DOF Discreto/Subsystem1 ==
  In1 : Inport
  Add : Sum
  Add1 : Sum
  Demux : Demux  Outputs=2
  Gain : Gain  Gain=CL  Multiplication=Matrix(K*u)
  Gain1 : Gain  Gain=AL  Multiplication=Matrix(K*u)
  Gain2 : Gain  Gain=DL  Multiplication=Matrix(K*u)
  Gain3 : Gain  Gain=BL  Multiplication=Matrix(K*u)
  Integrator : Integrator
  Terminator : Terminator
  YL : Outport
  Est_L : Outport  Port=2
  wires:
  Gain/1 -> Add/2
  Integrator/1 -> Gain/1, Est_L/1, Gain1/1
  Add1/1 -> Integrator/1
  Gain1/1 -> Add1/2
  Gain2/1 -> Add/1
  Gain3/1 -> Add1/1
  In1/1 -> Gain2/1, Gain3/1
  Add/1 -> Demux/1
  Demux/1 -> YL/1
  Demux/2 -> Terminator/1

== system controladorPaola/PID 2 DOF/Subsystem ==
  Input : Inport
  Add : Sum
  Constant : Constant  Value=[Ro, Lo, Kio, Kvo, Jmo, Jlo, Bmo, Blo, no, go, do, mo]
  Constant1 : Constant  Value=Vin0
  Constant2 : Constant  Value=[X10; X20; X30]
  Demux : Demux  Outputs=2
  Gain : Gain  Gain=DL  Multiplication=Matrix(K*u)
  Gain1 : Gain  Gain=CL  Multiplication=Matrix(K*u)
  Integrator : Integrator  InitialCondition=[X10; X20; X30]
  MATLAB Function : MATLAB Function  TreatAsAtomicUnit=on
  Subtract : Sum
  Subtract1 : Sum  Inputs=+-
  Output : Outport
  Output1 : Outport  Port=2
  Output2 : Outport  Port=3
  wires:
  Integrator/1 -> Subtract1/1, MATLAB Function/1(x)
  Add/1 -> MATLAB Function/2(PWM)
  Subtract1/1 -> Output1/1, Gain1/1
  MATLAB Function/1(dx) -> Integrator/1
  Constant1/1 -> Add/1
  Constant2/1 -> Subtract1/2
  Constant/1 -> MATLAB Function/3(parametros)
  Gain1/1 -> Subtract/1
  Gain/1 -> Subtract/2
  Input/1 -> Gain/1, Add/2
  Subtract/1 -> Demux/1
  Demux/1 -> Output/1
  Demux/2 -> Output2/1

== system controladorPaola/PID 2 DOF/Subsystem1 ==
  In1 : Inport
  Add : Sum
  Add1 : Sum
  Demux : Demux  Outputs=2
  Gain : Gain  Gain=CL  Multiplication=Matrix(K*u)
  Gain1 : Gain  Gain=AL  Multiplication=Matrix(K*u)
  Gain2 : Gain  Gain=DL  Multiplication=Matrix(K*u)
  Gain3 : Gain  Gain=BL  Multiplication=Matrix(K*u)
  Integrator : Integrator
  YL : Outport
  Est_L : Outport  Port=2
  Output : Outport  Port=3
  wires:
  Gain/1 -> Add/2
  Integrator/1 -> Gain/1, Est_L/1, Gain1/1
  Add1/1 -> Integrator/1
  Gain1/1 -> Add1/2
  Gain2/1 -> Add/1
  Gain3/1 -> Add1/1
  In1/1 -> Gain2/1, Gain3/1
  Add/1 -> Demux/1
  Demux/1 -> YL/1
  Demux/2 -> Output/1

== system controladorPaola/PID 2 DOF Discreto/Subsystem ==
  Input : Inport
  Add : Sum
  Constant : Constant  Value=[Ro, Lo, Kio, Kvo, Jmo, Jlo, Bmo, Blo, no, go, do, mo]
  Constant1 : Constant  Value=Vin0
  Constant2 : Constant  Value=[X10; X20; X30]
  Demux : Demux  Outputs=2
  Gain : Gain  Gain=DL  Multiplication=Matrix(K*u)
  Gain1 : Gain  Gain=CL  Multiplication=Matrix(K*u)
  Integrator : Integrator  InitialCondition=[X10; X20; X30]
  MATLAB Function : MATLAB Function  TreatAsAtomicUnit=on
  Subtract : Sum
  Subtract1 : Sum  Inputs=+-
  Output : Outport
  Output1 : Outport  Port=2
  Output2 : Outport  Port=3
  wires:
  Integrator/1 -> Subtract1/1, MATLAB Function/1(x)
  Add/1 -> MATLAB Function/2(PWM)
  Subtract1/1 -> Output1/1, Gain1/1
  MATLAB Function/1(dx) -> Integrator/1
  Constant1/1 -> Add/1
  Constant2/1 -> Subtract1/2
  Constant/1 -> MATLAB Function/3(parametros)
  Gain1/1 -> Subtract/1
  Gain/1 -> Subtract/2
  Input/1 -> Gain/1, Add/2
  Subtract/1 -> Demux/1
  Demux/1 -> Output/1
  Demux/2 -> Output2/1

== system controladorPaola/PID 2 DOF Discreto/Subsystem1 ==
  In1 : Inport
  Add : Sum
  Add1 : Sum
  Demux : Demux  Outputs=2
  Gain : Gain  Gain=CL  Multiplication=Matrix(K*u)
  Gain1 : Gain  Gain=AL  Multiplication=Matrix(K*u)
  Gain2 : Gain  Gain=DL  Multiplication=Matrix(K*u)
  Gain3 : Gain  Gain=BL  Multiplication=Matrix(K*u)
  Integrator : Integrator
  Terminator : Terminator
  YL : Outport
  Est_L : Outport  Port=2
  wires:
  Gain/1 -> Add/2
  Integrator/1 -> Gain/1, Est_L/1, Gain1/1
  Add1/1 -> Integrator/1
  Gain1/1 -> Add1/2
  Gain2/1 -> Add/1
  Gain3/1 -> Add1/1
  In1/1 -> Gain2/1, Gain3/1
  Add/1 -> Demux/1
  Demux/1 -> YL/1
  Demux/2 -> Terminator/1

== system controladorPaola/PID Cascada/Subsystem1 ==
  Input : Inport
  Add : Sum
  Constant : Constant  Value=[Ro, Lo, Kio, Kvo, Jmo, Jlo, Bmo, Blo, no, go, do, mo]
  Constant1 : Constant  Value=Vin0
  Constant2 : Constant  Value=[X10; X20; X30]
  Demux : Demux  Outputs=2
  Gain : Gain  Gain=DL  Multiplication=Matrix(K*u)
  Gain1 : Gain  Gain=CL  Multiplication=Matrix(K*u)
  Integrator : Integrator  InitialCondition=[X10; X20; X30]
  MATLAB Function : MATLAB Function  TreatAsAtomicUnit=on
  Subtract : Sum
  Subtract1 : Sum  Inputs=+-
  Output : Outport
  Output1 : Outport  Port=2
  Output2 : Outport  Port=3
  wires:
  Integrator/1 -> Subtract1/1, MATLAB Function/1(x)
  Add/1 -> MATLAB Function/2(PWM)
  Subtract1/1 -> Output1/1, Gain1/1
  MATLAB Function/1(dx) -> Integrator/1
  Constant1/1 -> Add/1
  Constant2/1 -> Subtract1/2
  Constant/1 -> MATLAB Function/3(parametros)
  Gain1/1 -> Subtract/1
  Gain/1 -> Subtract/2
  Input/1 -> Gain/1, Add/2
  Subtract/1 -> Demux/1
  Demux/1 -> Output/1
  Demux/2 -> Output2/1

== system controladorPaola/PID Cascada/Subsystem2 ==
  In1 : Inport
  Add : Sum
  Add1 : Sum
  Demux : Demux  Outputs=2
  Gain : Gain  Gain=CL  Multiplication=Matrix(K*u)
  Gain1 : Gain  Gain=AL  Multiplication=Matrix(K*u)
  Gain2 : Gain  Gain=DL  Multiplication=Matrix(K*u)
  Gain3 : Gain  Gain=BL  Multiplication=Matrix(K*u)
  Integrator : Integrator
  YL : Outport
  Est_L : Outport  Port=2
  Output : Outport  Port=3
  wires:
  Gain/1 -> Add/2
  Integrator/1 -> Gain/1, Est_L/1, Gain1/1
  Add1/1 -> Integrator/1
  Gain1/1 -> Add1/2
  Gain2/1 -> Add/1
  Gain3/1 -> Add1/1
  In1/1 -> Gain2/1, Gain3/1
  Add/1 -> Demux/1
  Demux/1 -> YL/1
  Demux/2 -> Output/1

== system controladorPaola/PID Cascada Discreto/Subsystem1 ==
  Input : Inport
  Add : Sum
  Constant : Constant  Value=[Ro, Lo, Kio, Kvo, Jmo, Jlo, Bmo, Blo, no, go, do, mo]
  Constant1 : Constant  Value=Vin0
  Constant2 : Constant  Value=[X10; X20; X30]
  Demux : Demux  Outputs=2
  Gain : Gain  Gain=DL  Multiplication=Matrix(K*u)
  Gain1 : Gain  Gain=CL  Multiplication=Matrix(K*u)
  Integrator : Integrator  InitialCondition=[X10; X20; X30]
  MATLAB Function : MATLAB Function  TreatAsAtomicUnit=on
  Subtract : Sum
  Subtract1 : Sum  Inputs=+-
  Output : Outport
  Output1 : Outport  Port=2
  Output2 : Outport  Port=3
  wires:
  Integrator/1 -> Subtract1/1, MATLAB Function/1(x)
  Add/1 -> MATLAB Function/2(PWM)
  Subtract1/1 -> Output1/1, Gain1/1
  MATLAB Function/1(dx) -> Integrator/1
  Constant1/1 -> Add/1
  Constant2/1 -> Subtract1/2
  Constant/1 -> MATLAB Function/3(parametros)
  Gain1/1 -> Subtract/1
  Gain/1 -> Subtract/2
  Input/1 -> Gain/1, Add/2
  Subtract/1 -> Demux/1
  Demux/1 -> Output/1
  Demux/2 -> Output2/1

== system controladorPaola/PID Cascada Discreto/Subsystem2 ==
  In1 : Inport
  Add : Sum
  Add1 : Sum
  Demux : Demux  Outputs=2
  Gain : Gain  Gain=CL  Multiplication=Matrix(K*u)
  Gain1 : Gain  Gain=AL  Multiplication=Matrix(K*u)
  Gain2 : Gain  Gain=DL  Multiplication=Matrix(K*u)
  Gain3 : Gain  Gain=BL  Multiplication=Matrix(K*u)
  Integrator : Integrator
  YL : Outport
  Est_L : Outport  Port=2
  Output : Outport  Port=3
  wires:
  Gain/1 -> Add/2
  Integrator/1 -> Gain/1, Est_L/1, Gain1/1
  Add1/1 -> Integrator/1
  Gain1/1 -> Add1/2
  Gain2/1 -> Add/1
  Gain3/1 -> Add1/1
  In1/1 -> Gain2/1, Gain3/1
  Add/1 -> Demux/1
  Demux/1 -> YL/1
  Demux/2 -> Output/1

== system controladorPaola/Seg. Estados/Subsystem1 ==
  In1 : Inport
  Add : Sum
  Add1 : Sum
  Gain : Gain  Gain=CL  Multiplication=Matrix(K*u)
  Gain1 : Gain  Gain=AL  Multiplication=Matrix(K*u)
  Gain2 : Gain  Gain=DL  Multiplication=Matrix(K*u)
  Gain3 : Gain  Gain=BL  Multiplication=Matrix(K*u)
  Integrator : Integrator
  YL : Outport
  Est_L : Outport  Port=2
  wires:
  Gain/1 -> Add/2
  Integrator/1 -> Gain/1, Est_L/1, Gain1/1
  Add1/1 -> Integrator/1
  Gain1/1 -> Add1/2
  Gain2/1 -> Add/1
  Gain3/1 -> Add1/1
  Add/1 -> YL/1
  In1/1 -> Gain2/1, Gain3/1

== system controladorPaola/Seg. Estados/Subsystem2 ==
  Input : Inport
  Add : Sum
  Constant : Constant  Value=[Ro,Lo,Kio, Kvo, Jmo, Jlo, Bmo, Blo, no, go, do, mo]
  Constant1 : Constant  Value=Vin0
  Constant2 : Constant  Value=[X10; X20]
  Gain1 : Gain  Gain=CL  Multiplication=Matrix(K*u)
  Integrator : Integrator  InitialCondition=[X10; X20]
  MATLAB Function : MATLAB Function  TreatAsAtomicUnit=on
  Subtract1 : Sum  Inputs=+-
  Output : Outport
  Est : Outport  Port=2
  wires:
  Add/1 -> MATLAB Function/2(PWM)
  Constant2/1 -> Subtract1/2
  Constant1/1 -> Add/1
  Input/1 -> Add/2
  MATLAB Function/1(dx) -> Integrator/1
  Constant/1 -> MATLAB Function/3(parametros)
  Integrator/1 -> Subtract1/1, MATLAB Function/1(x)
  Subtract1/1 -> Est/1, Gain1/1
  Gain1/1 -> Output/1

== system controladorPaola/Seg. Estados 2DOF Discreto/Subsystem1 ==
  In1 : Inport
  Add : Sum
  Add1 : Sum
  Gain : Gain  Gain=CL  Multiplication=Matrix(K*u)
  Gain1 : Gain  Gain=AL  Multiplication=Matrix(K*u)
  Gain2 : Gain  Gain=DL  Multiplication=Matrix(K*u)
  Gain3 : Gain  Gain=BL  Multiplication=Matrix(K*u)
  Integrator : Integrator
  YL : Outport
  Est_L : Outport  Port=2
  wires:
  Gain/1 -> Add/2
  Integrator/1 -> Gain/1, Est_L/1, Gain1/1
  Add1/1 -> Integrator/1
  Gain1/1 -> Add1/2
  Gain2/1 -> Add/1
  Gain3/1 -> Add1/1
  Add/1 -> YL/1
  In1/1 -> Gain2/1, Gain3/1

== system controladorPaola/Seg. Estados 2DOF Discreto/Subsystem2 ==
  Input : Inport
  Add : Sum
  Constant : Constant  Value=[Ro,Lo,Kio, Kvo, Jmo, Jlo, Bmo, Blo, no, go, do, mo]
  Constant1 : Constant  Value=Vin0
  Constant2 : Constant  Value=[X10; X20;X30]
  Gain1 : Gain  Gain=CL  Multiplication=Matrix(K*u)
  Integrator : Integrator  InitialCondition=[X10; X20;X30]
  MATLAB Function : MATLAB Function  TreatAsAtomicUnit=on
  Subtract1 : Sum  Inputs=+-
  Output : Outport
  Est : Outport  Port=2
  wires:
  Add/1 -> MATLAB Function/2(PWM)
  Constant2/1 -> Subtract1/2
  Constant1/1 -> Add/1
  Input/1 -> Add/2
  MATLAB Function/1(dx) -> Integrator/1
  Constant/1 -> MATLAB Function/3(parametros)
  Integrator/1 -> Subtract1/1, MATLAB Function/1(x)
  Subtract1/1 -> Est/1, Gain1/1
  Gain1/1 -> Output/1

== system controladorPaola/Seg. Estados Desacop-/Subsystem1 ==
  In1 : Inport
  Add : Sum
  Add1 : Sum
  Gain : Gain  Gain=CL  Multiplication=Matrix(K*u)
  Gain1 : Gain  Gain=AL  Multiplication=Matrix(K*u)
  Gain2 : Gain  Gain=DL  Multiplication=Matrix(K*u)
  Gain3 : Gain  Gain=BL  Multiplication=Matrix(K*u)
  Integrator : Integrator
  YL : Outport
  Est_L : Outport  Port=2
  wires:
  Gain/1 -> Add/2
  Integrator/1 -> Gain/1, Est_L/1, Gain1/1
  Add1/1 -> Integrator/1
  Gain1/1 -> Add1/2
  Gain2/1 -> Add/1
  Gain3/1 -> Add1/1
  Add/1 -> YL/1
  In1/1 -> Gain2/1, Gain3/1

== system controladorPaola/Seg. Estados Desacop-/Subsystem2 ==
  Input : Inport
  Add : Sum
  Constant : Constant  Value=[Ro,Lo,Kio, Kvo, Jmo, Jlo, Bmo, Blo, no, go, do, mo]
  Constant1 : Constant  Value=Vin0
  Constant2 : Constant  Value=[X10; X20;X30]
  Gain1 : Gain  Gain=CL  Multiplication=Matrix(K*u)
  Integrator : Integrator  InitialCondition=[X10; X20;X30]
  MATLAB Function : MATLAB Function  TreatAsAtomicUnit=on
  Subtract1 : Sum  Inputs=+-
  Output : Outport
  Est : Outport  Port=2
  wires:
  Add/1 -> MATLAB Function/2(PWM)
  Constant2/1 -> Subtract1/2
  Constant1/1 -> Add/1
  Input/1 -> Add/2
  MATLAB Function/1(dx) -> Integrator/1
  Constant/1 -> MATLAB Function/3(parametros)
  Integrator/1 -> Subtract1/1, MATLAB Function/1(x)
  Subtract1/1 -> Est/1, Gain1/1
  Gain1/1 -> Output/1

== system controladorPaola/Seg. Estados Desacop-/Subsystem3 ==
  U : Inport
  Y : Inport  Port=2
  Add6 : Sum
  Add7 : Sum
  Add8 : Sum
  Add9 : Sum  Inputs=+-
  Gain10 : Gain  Gain=CL  Multiplication=Matrix(K*u)
  Gain11 : Gain  Gain=DL  Multiplication=Matrix(K*u)
  Gain13 : Gain  Gain=L  Multiplication=Matrix(K*u)
  Gain8 : Gain  Gain=BL  Multiplication=Matrix(K*u)
  Gain9 : Gain  Gain=AL  Multiplication=Matrix(K*u)
  Integrator3 : Integrator
  Estados : Outport  VectorParamsAs1DForOutWhenUnconnected=off
  wires:
  Gain9/1 -> Add6/2
  Add6/1 -> Integrator3/1
  Integrator3/1 -> Gain9/1, Estados/1, Gain10/1
  Y/1 -> Add9/1
  Add7/1 -> Add9/2
  Add8/1 -> Add6/1
  Add9/1 -> Gain13/1
  Gain13/1 -> Add8/2
  Gain11/1 -> Add7/1
  Gain10/1 -> Add7/2
  Gain8/1 -> Add8/1
  U/1 -> Gain11/1, Gain8/1

== system controladorPaola/Seg. Estados Desacop-/Subsystem4 ==
  U : Inport
  Y : Inport  Port=2
  Add6 : Sum
  Add7 : Sum
  Add8 : Sum
  Add9 : Sum  Inputs=+-
  Gain10 : Gain  Gain=CL  Multiplication=Matrix(K*u)
  Gain11 : Gain  Gain=DL  Multiplication=Matrix(K*u)
  Gain13 : Gain  Gain=L  Multiplication=Matrix(K*u)
  Gain8 : Gain  Gain=BL  Multiplication=Matrix(K*u)
  Gain9 : Gain  Gain=AL  Multiplication=Matrix(K*u)
  Integrator3 : Integrator
  Estados : Outport  VectorParamsAs1DForOutWhenUnconnected=off
  wires:
  Gain9/1 -> Add6/2
  Add6/1 -> Integrator3/1
  Integrator3/1 -> Gain9/1, Estados/1, Gain10/1
  Y/1 -> Add9/1
  Add7/1 -> Add9/2
  Add8/1 -> Add6/1
  Add9/1 -> Gain13/1
  Gain13/1 -> Add8/2
  Gain11/1 -> Add7/1
  Gain10/1 -> Add7/2
  Gain8/1 -> Add8/1
  U/1 -> Gain11/1, Gain8/1
